simulink model "prob17_b"  (R2013a)
settings: Solver=ode45  StartTime=0.0  StopTime=10.0  RelTol=1e-3
settings Model: Creator=Suddenlink  LastModifiedBy=Suddenlink

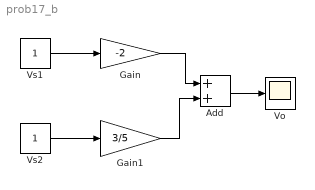
== system prob17_b ==
  Add : Sum
  Gain : Gain  Gain=-2
  Gain1 : Gain  Gain=3/5
  Vo : Scope
  Vs1 : Constant
  Vs2 : Constant
  wires:
  Vs1/1 -> Gain/1
  Vs2/1 -> Gain1/1
  Gain1/1 -> Add/2
  Gain/1 -> Add/1
  Add/1 -> Vo/1
